simulink model "untitled"  (R2017a)
settings: Solver=VariableStepAuto  StartTime=0.0  StopTime=15  RelTol=1e-3
settings Model: Creator=lenovo  LastModifiedBy=lenovo

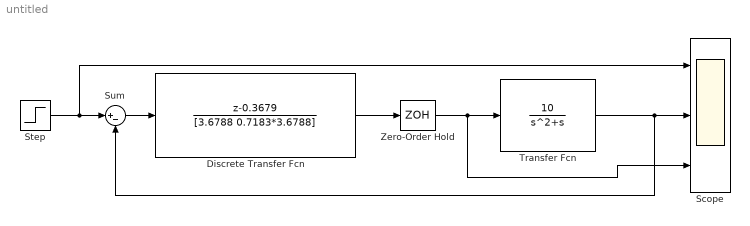
== system untitled ==
  Discrete Transfer Fcn : DiscreteTransferFcn  Numerator=[1 -0.3679]  Denominator=[3.6788 0.7183*3.6788]
  Scope : Scope  NumInputPorts=3
  Step : Step  SampleTime=0
  Sum : Sum  Inputs=|+-
  Transfer Fcn : TransferFcn  Numerator=[10]  Denominator=[1 1 0]
  Zero-Order Hold : ZeroOrderHold
  wires:
  Zero-Order Hold/1 -> Transfer Fcn/1, Scope/3
  Discrete Transfer Fcn/1 -> Zero-Order Hold/1
  Step/1 -> Scope/1, Sum/1
  Transfer Fcn/1 -> Sum/2, Scope/2
  Sum/1 -> Discrete Transfer Fcn/1
